simulink model "new68bus_opal"  (R2019b)
settings: Solver=ode4  StartTime=0.0  StopTime=30  FixedStep=Ts  RelTol=1e-3
PreLoadFcn:
  | PSSMODEL=1;
  | LPSS=0;
  | WAPSS=0;
  | WAPSS2=0;
  | Ts=50e-5;
InitFcn:
  | PSSMODEL=1;
  | LPSS=0;
  | WAPSS=0;
  | WAPSS2=0;
  | Ts=50e-5;
  | 
  | % Required data to 68 Bus benchmark
  | % clear
  | % clc
  | % Definition for the columns
  | % system base =100 MVA
  | 
  | %% Line data Format (line)
  | % All values are given on the same system base MVA
  | % 1: From bus
  | % 2: To bus
  | % 3: Resistance (pu)
  | % 4: Reactance  (pu)
  | % 5: Charge     (pu)
  | % 6: Transformer Tap Amplitute
  | % 7: base MVA
  | % 8: Nomonal Voltage (KV)
  | 
  | %1   2    3        4       5       6        7      8
  | line=[...
  | 1	54	0	     0.0181	  0	      1.025     100    13.8
  | 2	58	0	     0.025	  0	      1.070     100    13.8
  | 3	62	0	     0.02	  0	      1.070     100    13.8
  | 4	19	0.0007	 0.0142	  0	      1.070     100    13.8
  | 5	20	0.0009	 0.018	  0	      1.009     100    13.8
  | 6	22	0	     0.0143	  0	      1.025     100    13.8
  | 7	23	0.0005	 0.0272	  0	      0         100    13.8
  | 8	25	0.0006	 0.0232	  0	      1.025     100    13.8
  | 9	29	0.0008	 0.0156   0	      1.025     100    13.8
  | 10	31	0	     0.026	  0	      1.04      100    13.8
  | 11	32	0	     0.013	  0	      1.04      100    13.8
  | 12	36	0	     0.0075	  0	      1.04      100    13.8
  | 13	17	0	     0.0033	  0	      1.04      100    13.8
  | 14	41	0	     0.0015	  0	      1         100    13.8
  | 15	42	0	     0.0015	  0	      1         100    13.8
  | 16	18	0	     0.003	  0	      1         100    13.8
  | 17	36	0.0005	 0.0045	  0.32	  0         100    138
  | 17	43	0.0005	 0.0276	  0	      0         100    138
  | 18	42	0.004	 0.06	  2.25    0         100    138
  | 18	49	0.0076	 0.1141	  1.16    0	        100    138
  | 18	50	0.0012	 0.0288	  2.06	  0         100    138
  | 20	19	0.0007	 0.0138	  0       1.06	    100    138
  | 19	68	0.0016	 0.0195	  0.304	  0         100    138
  | 21	22	0.0008	 0.014	  0.2565  0	        100    138
  | 21	68	0.0008	 0.0135	  0.2548  0	        100    138
  | 22	23	0.0006	 0.0096	  0.1846  0	        100    138
  | 23	24	0.0022	 0.035	  0.361	  0         100    138
  | 24	68	0.0003	 0.0059	  0.068	  0         100    138
  | 25	26	0.0032	 0.0323	  0.531	  0         100    138
  | 25	54	0.007	 0.0086	  0.146	  0         100    138
  | 26	27	0.0014	 0.0147	  0.2396  0	        100    138
  | 26	28	0.0043	 0.0474	  0.7802  0	        100    138
  | 26	29	0.0057	 0.0625	  1.029	  0         100    138
  | 27	37	0.0013	 0.0173	  0.3216  0	        100    138
  | 27	53	0.032	 0.32	  0.41	  0         100    138
  | 29	28	0.0014	 0.0151	  0.249	  0         100    138
  | 30	31	0.0013	 0.0187	  0.333	  0         100    138
  | 30	32	0.0024	 0.0288	  0.488	  0         100    138
  | 30	53	0.0008	 0.0074	  0.48	  0         100    138
  | 30	61	0.00095	 0.00915  0.58	  0         100    138
  | 31	38	0.0011	 0.0147	  0.247	  0         100    138
  | 31	53	0.0016	 0.0163	  0.25	  0         100    138
  | 32	33	0.0008	 0.0099	  0.168	  0         100    138
  | 33	34	0.0011	 0.0157	  0.202	  0         100    138
  | 33	38	0.0036	 0.0444	  0.693	  0         100    138
  | 34	35	0.0001	 0.0074	  0	      0.946     100    138
  | 34	36	0.0033	 0.0111	  1.45	  0         100    138
  | 35	45	0.0007	 0.0175	  1.39	  0         100    138
  | 36	61	0.0011	 0.0098	  0.68	  0         100    138
  | 37	52	0.0007	 0.0082	  0.1319  0	        100    138
  | 37	68	0.0007	 0.0089	  0.1342  0	        100    138
  | 38	46	0.0022	 0.0284	  0.43	  0         100    138
  | 39	44	0	     0.0411	  0	      0         100    138
  | 39	45	0	     0.0839	  0	      0         100    138
  | 40	41	0.006	 0.084	  3.15	  0         100    138
  | 40	48	0.002	 0.022	  1.28	  0         100    138
  | 41	42	0.004	 0.06	  2.25	  0         100    138
  | 43	44	0.0001	 0.0011	  0	      0         100    138
  | 44	45	0.0025	 0.073	  0	      0         100    138
  | 45	51	0.0004	 0.0105	  0.72	  0         100    138
  | 46	49	0.0018	 0.0274	  0.27	  0         100    138
  | 47	48	0.00125	 0.0134	  0.8	  0         100    138
  | 47	53	0.0013	 0.0188	  1.31	  0         100    138
  | 50	51	0.0009	 0.0221	  1.62	  0         100    138
  | 52	55	0.0011	 0.0133	  0.2138  0	        100    138
  | 53	54	0.0035	 0.0411	  0.6987  0	        100    138
  | 54	55	0.0013	 0.0151	  0.2572  0	        100    138
  | 55	56	0.0013	 0.0213	  0.2214  0	        100    138
  | 56	57	0.0008	 0.0128	  0.1342  0	        100    138
  | 56	66	0.0008	 0.0129	  0.1382  0	        100    138
  | 57	58	0.0002	 0.0026	  0.0434  0	        100    138
  | 57	60	0.0008	 0.0112	  0.1476  0	        100    138
  | 58	59	0.0006	 0.0092	  0.113	  0         100    138
  | 58	63	0.0007	 0.0082	  0.1389  0	        100    138
  | 59	60	0.0004	 0.0046	  0.078	  0         100    138
  | 60	61	0.0023	 0.0363	  0.3804  0	        100    138
  | 62	63	0.0004	 0.0043	  0.0729  0	        100    138
  | 62	65	0.0004	 0.0043	  0.0729  0	        100    138
  | 63	64	0.0016	 0.0435	  0	      1.06      100    138
  | 65	64	0.0016	 0.0435	  0	      1.06      100    138
  | 65	66	0.0009	 0.0101	  0.1723  0 	    100    138
  | 66	67	0.0018	 0.0217	  0.366	  0         100    138
  | 67	68	0.0009	 0.0094   0.171   0         100   138 ];
  | 
  | 
  | 
  | %% Power System Stabilizer Format (MB)
  | % Applied power system stabilizer is MBPSS with simplified settings
  | % Note: All machines use MBPSS with same configuration
  | % 1: Global gain (G)
  | % 2: Frequency of low frequency band (FL) Hz
  | % 3: Gain of low frequency band (KL)
  | % 4: Frequency of intermediate frequency band (FI) Hz
  | % 5: Gain of intermediate frequency band (KI)
  | % 6: Frequency of high frequency band (FH) Hz
  | % 7: Gain of high frequency band (KH)
  | %   1    2  3     4   5      6  7
  | MB=[1   0.2 30   1.25 40    12 160];
  | 
  | %% Excitation System format (AVR_Data)
  | % All machines use IEEE type 1 synchronous machine voltage regulator combined to an exciter
  | % 1. Low pass filter time constant (Tr) sec
  | % 2. Regulator gain (Ka)
  | % 3. regulator time constant (Ta) sec
  | % 4. Lead-lag compensator time constant (Tb) sec
  | % 5. Lead-lag compensator time constant (Tc) sec
  | % 6. Terminal voltage (pu)
  | % 7. Lower limit for regulator output (Emin)
  | % 8. Upper limit for regulator output (Emax)
  | %     1    2      3      4     5     6       7    8
  |   AVR_Data=[...
  |     0.01  200    0.015   10    1    1.03    -5    5
  |     0.01  200    0.015   10    1    1.03    -5    5
  |     0.01  200    0.015   10    1    1.03    -5    5
  |     0.01  200    0.015   10    1    1.03    -5    5
  |     0.01  200    0.015   10    1    1.03    -5    5
  |     0.01  200    0.015   10    1    1.03    -5    5
  |     0.01  200    0.015   10    1    1.03    -5    5
  |     0.01  200    0.015   10    1    1.03    -5    5
  |     0.01  200    0.015   10    1    1.03    -5    5
  |     0.01  200    0.015   10    1    1.03    -5    5
  |     0.01  200    0.015   10    1    1.03    -5    5
  |     0.01  200    0.015   10    1    1.03    -5    5
  |     0.01  200    0.015   10    1    1.03    -5    5
  |     0.01  200    0.015   10    1    1.03    -5    5
  |     0.01  200    0.015   10    1    1.03    -5    5
  |     0.01  200    0.015   10    1    1.03    -5    5];
  | 
  | C0=829.7e-9;
  | L0=3.220e-3;
  | R0=1;
  | Ns=120*60/(2); %Nominal speed of synchronous machines
  | s=10;
  | 
  | %% Machine Data Format (mac_con)
  | % 1.  Machine Number
  | % 2.  Bus Number
  | % 3.  Base MVA
  | % 4.  Leakage Reactance x_l(pu)
  | % 5.  Resistance r_a(pu)
  | % 6.  d-axis sychronous reactance x_d(pu)
  | % 7.  d-axis transient reactance x'_d(pu)
  | % 8.  d-axis subtransient reactance x"_d(pu)
  | % 9.  d-axis open-circuit time constant T'_do(sec),
  | % 10. d-axis open-circuit subtransient time constant T"_do(sec)
  | % 11. q-axis sychronous reactance x_q(pu)
  | % 12. q-axis transient reactance x'_q(pu)
  | % 13. q-axis subtransient reactance x"_q(pu)
  | % 14. q-axis open-circuit time constant T'_qo(sec)
  | % 15. q-axis open circuit subtransient time constant % T"_qo(sec)
  | % 16. inertia constant H(sec)
  | % 17. damping coefficient d_o(pu)
  | % 18. dampling coefficient d_1(pu)
  | % 19. bus number
  | % Note: all the following machines use sub-transient model
  | % 1  2     3      4      5     6     7    8      9    10    11    12    13    14    15    16    17    18  19
  | mac_con = [ 01 01 100 0.0125 0.0 0.1 0.031 0.025 10.2 0.05 0.069 0.0416667 0.025 1.5 0.035 42. 0 0 01 0 0; 02 02 100 0.035 0.0 0.295 0.0697 0.05 6.56 0.05 0.282 0.0933333 0.05 1.5 0.035 30.2 0 0 02 0 0; 03 03 100 0.0304 0.0 0.2495 0.0531 0.045 5.7 0.05 0.237 0.0714286 0.045 1.5 0.035 35.8 0 0 03 0 0; 04 04 100 0.0295 0.0 0.262 0.0436 0.035 5.69 0.05 0.258 0.0585714 0.035 1.5 0.035 28.6 0 0 04 0 0; 05 05 100 0.027 0.0 0.33 0.066 0.05 5.4 0.05 0.31 0.0883333 0.05 0.44 0.035 26. 0 0 05 0 0; 06 06 100 0.0224 0.0 0.254 0.05 0.04 7.3 0.05 0.241 0.0675000 0.04 0.4 0.035 34.8 0 0 06 0 0; 07 07 100 0.0322 0.0 0.295 0.049 0.04 5.66 0.05 0.292 0.0666667 0.04 1.5 0.035 26.4 0 0 07 0 0; 08 08 100 0.028 0.0 0.29 0.057 0.045 6.7 0.05 0.280 0.0766667 0.045 0.41 0.035 24.3 0 0 08 0 0; 09 09 100 0.0298 0.0 0.2106 0.057 0.045 4.79 0.05 0.205 0.0766667 0.045 1.96 0.035 34.5 0 0 09 0 0; 10 10 100 0.0199 0.0 0.169 0.0457 0.04 9.37 0.05 0.115 0.0615385 0.04 1.5 0.035 31.0 0 0 10 0 0; 11 11 100 0.0103 0.0 0.128 0.018 0.012 4.1 0.05 0.123 0.0241176 0.012 1.5 0.035 28.2 0 0 11 0 0; 12 12 100 0.022 0.0 0.101 0.031 0.025 7.4 0.05 0.095 0.0420000 0.025 1.5 0.035 92.3 0 0 12 0 0; 13 13 200 0.0030 0.0 0.0296 0.0055 0.004 5.9 0.05 0.0286 0.0074000 0.004 1.5 0.035 248.0 0 0 13 0 0; 14 14 100 0.0017 0.0 0.018 0.00285 0.0023 4.1 0.05 0.0173 0.0037931 0.0023 1.5 0.035 300.0 0 0 14 0 0; 15 15 100 0.0017 0.0 0.018 0.00285 0.0023 4.1 0.05 0.0173 0.0037931 0.0023 1.5 0.035 300.0 0 0 15 0 0; 16 16 200 0.0041 0.0 0.0356 0.0071 0.0055 7.8 0.05 0.0334 0.0095000 0.0055 1.5 0.035 225.0 0 0 16 0 0; ] ;
  | 
  | p0=[250/200 545/200 650/200 632/200 505/200 700/200 560/200 540/200 800/200 500/200 1000/200 1350/200 3591/6000 1785/3000 1000/3000 3379.57/6000];%'./1000;%Active Power Generation of PV units
  | Pn(1:16,1)=1; % Nominal Power
  | % PSSModel=1;%1:No pSS //1:MB
  | %% Bus data (Bus)
  | % 1. Bus number
  | % 2. Nominal phase-phase voltage
  | %    1    2
  | Bus = [ ...
  | 1	13.8
  | 2	13.8
  | 3	13.8
  | 4	13.8
  | 5	13.8
  | 6	13.8
  | 7	13.8
  | 8	13.8
  | 9	13.8
  | 10	13.8
  | 11	13.8
  | 12	13.8
  | 13	13.8
  | 14	13.8
  | 15	13.8
  | 16	13.8
  | 17	138
  | 18	138
  | 19	138
  | 20	138
  | 21	138
  | 22	138
  | 23	138
  | 24	138
  | 25	138
  | 26	138
  | 27	138
  | 28	138
  | 29	138
  | 30	138
  | 31	138
  | 32	138
  | 33	138
  | 34	138
  | 35	138
  | 36	138
  | 37	138
  | 38	138
  | 39	138
  | 40	138
  | 41	138
  | 42	138
  | 43	138
  | 44	138
  | 45	138
  | 46	138
  | 47	138
  | 48	138
  | 49	138
  | 50	138
  | 51	138
  | 52	138
  | 53	138
  | 54	138
  | 55	138
  | 56	138
  | 57	138
  | 58	138
  | 59	138
  | 60	138
  | 61	138
  | 62	138
  | 63	138
  | 64	138
  | 65	138
  | 66	138
  | 67	138
  | 68	138];
  | 
  |    zbase=(line(:,8).^2)./line(:,7);
  |    line(:,3)=line(:,3).*zbase;
  |    line(:,4)=line(:,4).*zbase/(120*pi);
  |    line(:,5)=line(:,5)./zbase/(120*pi);
  | 
  | %PSSMODEL=1;
undefined symbols (not defined in the file or in its folder): D1, Delta, I, Left, Right, type, V
libraries: powerlib x359, artemis x26, sps_avr x16, powerlib_meascontrol x5, rtlab x1
(part 1 of 8)
settings Model: ARTEMISmethode_block_infos=$$__separator__$$new68bus_opal/ARTEMIS Guide$$__separator__$$  Creator=rubai  LastModifiedBy=shamim

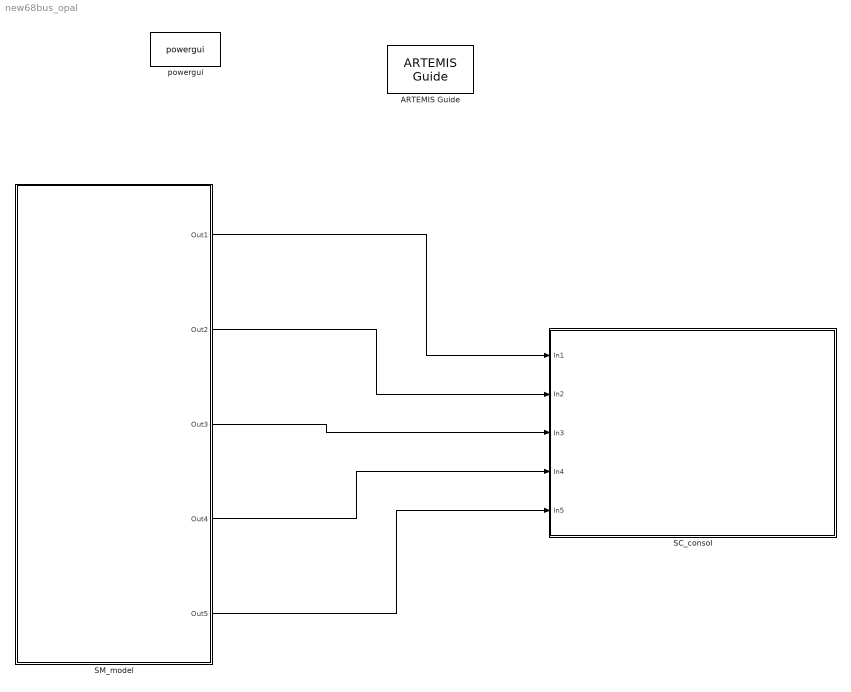
== system new68bus_opal ==
  ARTEMIS Guide : artemis/ARTEMIS/ARTEMIS Guide  Tag=art7.5  Description=New ARTEMiS block v 7.5b (R2015b+)  lock=on  Ts=Ts  ssn=on  opt=art5  dyna=off  nb_perm=4  RT_fullcomp=off  ssn_itvc=off  ssn_ivic=off  ssn_ext=off  ssn_solver=Art5  iter_type=iSWITCH and iMOV only (default)  ssn_ImpulseLoopBlockedStateUpdate=5  ssn_mov_iter_number=5  ssn_switch_iter_number=3  ssn_lu_or_ldlt=LU (more robust)  ssn_nib_type_verify=off  ssn_use_lu=on  ssn_use_ldlt=off  ssn_impulse=on  ssn_quasimpulse=off  ssn_impulse_loop=5  paraExtinctionThy=off  Thy_Impulse=on  dtc=Off  dtc_opt=normal  ao=off  simtype=off  ct_mac=off  lin_mov=off  lsp=[0.001 2]  spike_skip=Disabled  dtc_extra=1  dtc_sws=normal  dtc_pied=0.5  SPSRulesBlock=SPSRules  tre=off  ctmm=off  LF=off  dpl_type=ARTEMiS DPL  rlc_type=off  custom_type=off  para=on  ssn_full_iteration=off
  SC_consol : Subsystem
  SM_model : Subsystem
  powergui : powerlib/powergui  Priority=1  SimulationMode=Discrete  SampleTime=Ts  frequency=60  Iterations=50  frequencyindice=60  Pbase=100e6  ErrMax=1e-4  UnitsV=kV  UnitsW=MW  buscounter=0  FunctionMessages=off  echomessages=off  EnableUseOfTLC=off  CurrentSourceSwitches=off  DisableSnubberDevices=off  DisableRonSwitches=off  DisableVfSwitches=off  DisplayEquations=off  AutomaticDiscreteSolvers=on  SolverType=Tustin/Backward Euler (TBE)  Interpol=off  ExternalGateDelay=off  methode=off  Ts=100  x0status=blocks  SPID=on  SwTol=0  HookPort=off  NonlinearTolerance=1e-4  nMaxIteration=100  ContinueOnMaxIteration=off  RestoreLinks=warning  ResistiveCurrentMeasurement=off  Frange=[0:2:500]  Ylog=off  Xlog=on  ShowGrid=off  save=off  variable=ZData  structure=0  ZoomFFT=off  StartTime=0.0  cycles=1  DisplayStyle=1  fundamental=60  FreqAxis=off  MaxFrequency=1000  frequencyindicesteady=1  RmsSteady=1  display=off
      settings: SourceProductName=Simscape Electrical
  wires:
  SM_model/1(Out1) -> SC_consol/1(In1)
  SM_model/2(Out2) -> SC_consol/2(In2)
  SM_model/3(Out3) -> SC_consol/3(In3)
  SM_model/4(Out4) -> SC_consol/4(In4)
  SM_model/5(Out5) -> SC_consol/5(In5)

== system new68bus_opal/SC_consol ==
  In1 : Inport
  In2 : Inport  Port=2
  In3 : Inport  Port=3
  In4 : Inport  Port=4
  In5 : Inport  Port=5
  Display : Display
  OpComm : rtlab/OpComm  nbport=5  groupe_acq=1  subsys_rate=0  st=0  Synchronization=off  Interpolation=off  Threshold=1.0  Missed_Data=off  Sim_Time=off  Samples=off  dynSigOut=off  from_console=0  warning_done=off  writeOpCommFile=off  Offset=off
      settings: SourceProductName=RT-LAB
  Scope{,1..4} (5 alike) : Scope
  wires:
  In2/1 -> OpComm/2
  In5/1 -> OpComm/5
  In3/1 -> OpComm/3
  OpComm/1 -> Scope/1
  OpComm/2 -> Display/1, Scope1/1
  OpComm/3 -> Scope2/1
  In4/1 -> OpComm/4
  OpComm/5 -> Scope4/1
  OpComm/4 -> Scope3/1
  In1/1 -> OpComm/1

== system new68bus_opal/SM_model ==
  20-1 : powerlib/Elements/Three-Phase PI Section Line  LConnTagsString=a|b|c  RConnTagsString=A|B|C  Frequency=60  Resistances=[line(20,3) 3*line(20,3)]  Inductances=[line(20,4) 3*line(20,4)]  Capacitances=[line(20,5) line(20,5)/3]  Length=1
      settings: SourceProductName=Simscape Electrical
  21-1 : powerlib/Elements/Three-Phase PI Section Line  LConnTagsString=a|b|c  RConnTagsString=A|B|C  Frequency=60  Resistances=[line(21,3) 3*line(21,3)]  Inductances=[line(21,4) 3*line(21,4)]  Capacitances=[line(21,5) line(21,5)/3]  Length=1
      settings: SourceProductName=Simscape Electrical
  34-1 : powerlib/Elements/Three-Phase PI Section Line  LConnTagsString=a|b|c  RConnTagsString=A|B|C  Frequency=60  Resistances=[line(34,3) 3*line(34,3)]  Inductances=[line(34,4) 3*line(34,4)]  Capacitances=[line(34,5) line(34,5)/3]  Length=1
      settings: SourceProductName=Simscape Electrical
  39-1 : powerlib/Elements/Three-Phase PI Section Line  LConnTagsString=a|b|c  RConnTagsString=A|B|C  Frequency=60  Resistances=[line(39,3) 3*line(39,3)]  Inductances=[line(39,4) 3*line(39,4)]  Capacitances=[line(39,5) line(39,5)/3]  Length=1
      settings: SourceProductName=Simscape Electrical
  42-1 : powerlib/Elements/Three-Phase PI Section Line  LConnTagsString=a|b|c  RConnTagsString=A|B|C  Frequency=60  Resistances=[line(42,3) 3*line(42,3)]  Inductances=[line(42,4) 3*line(42,4)]  Capacitances=[line(42,5) line(42,5)/3]  Length=1
      settings: SourceProductName=Simscape Electrical
  51-1 : powerlib/Elements/Three-Phase PI Section Line  LConnTagsString=a|b|c  RConnTagsString=A|B|C  Frequency=60  Resistances=[line(51,3) 3*line(51,3)]  Inductances=[line(51,4) 3*line(51,4)]  Capacitances=[line(51,5) line(51,5)/3]  Length=1
      settings: SourceProductName=Simscape Electrical
  62-1 : powerlib/Elements/Three-Phase PI Section Line  LConnTagsString=a|b|c  RConnTagsString=A|B|C  Frequency=60  Resistances=[line(62,3) 3*line(62,3)]  Inductances=[line(62,4) 3*line(62,4)]  Capacitances=[line(62,5) line(62,5)/3]  Length=1
      settings: SourceProductName=Simscape Electrical
  67-1 : powerlib/Elements/Three-Phase PI Section Line  LConnTagsString=a|b|c  RConnTagsString=A|B|C  Frequency=60  Resistances=[line(67,3) 3*line(67,3)]  Inductances=[line(67,4) 3*line(67,4)]  Capacitances="[line(67,5)  line(67,5)/3]"  Length=1
      settings: SourceProductName=Simscape Electrical
  76-1 : powerlib/Elements/Three-Phase PI Section Line  LConnTagsString=a|b|c  RConnTagsString=A|B|C  Frequency=60  Resistances=[line(76,3) 3*line(76,3)]  Inductances=[line(76,4) 3*line(76,4)]  Capacitances=[line(76,5) line(76,5)/3]  Length=1
      settings: SourceProductName=Simscape Electrical
  83-1 : powerlib/Elements/Three-Phase PI Section Line  LConnTagsString=a|b|c  RConnTagsString=A|B|C  Frequency=60  Resistances=[line(83,3) 3*line(83,3)]  Inductances=[line(83,4) 3*line(83,4)]  Capacitances=[line(83,5) line(83,5)/3]  Length=1
      settings: SourceProductName=Simscape Electrical
  "Bus Voltages " : Subsystem  Commented=on
  PSS model : Constant  Value=PSSMODEL
  SSN Interface Block (3ph) : artemis/SSN/Nodal Interface Blocks/SSN Interface Block (3ph)  nb_phase=3  nb_port=2  p1_type=I-type(Left)  p2_type=I-type(Right)  p3_type=V-type(Left)  p4_type=V-type(Left)  p5_type=V-type(Left)  p6_type=V-type(Left)  p7_type=V-type(Left)  p8_type=V-type(Left)  p9_type=V-type(Left)  p10_type=V-type(Left)  p11_type=V-type(Left)  p12_type=V-type(Left)  p13_type=V-type(Left)  p14_type=V-type(Left)  p15_type=V-type(Left)  p16_type=V-type(Left)  I_port_shunt_resistance=1e9
  SSN group tag : artemis/SSN/SSN group tag  ssn_group_tag=ssn2a
  SSN group tag1 : artemis/SSN/SSN group tag  ssn_group_tag=ssn2b
  Subsystem : Subsystem
  area-1 : Subsystem
  area-2 : Subsystem
  area-3 : Subsystem
  area-4 : Subsystem
  "voltage measurement " : Subsystem
  Out1 : Outport
  Out2 : Outport  Port=2
  Out3 : Outport  Port=3
  Out4 : Outport  Port=4
  Out5 : Outport  Port=5
  tag scope: PSSmodel=global
  wires:
  "voltage measurement "/2(Output1) -> Out2/1
  "voltage measurement "/4(Output3) -> Out4/1
  "voltage measurement "/3(Output2) -> Out3/1
  PSS model/1 -> [PSSmodel]
  "voltage measurement "/1(Output) -> Out1/1
  "voltage measurement "/5(Output4) -> Out5/1
  connections:
  62-1/LConn3 -- area-3/RConn12
  62-1/RConn1 -- Subsystem/RConn5
  21-1/LConn3 -- area-4/RConn15
  51-1/LConn2 -- area-2/RConn6
  67-1/RConn1 -- area-3/RConn4
  83-1/LConn3 -- area-2/RConn3
  Subsystem/RConn2 -- 21-1/RConn2 -- 20-1/RConn2
  67-1/RConn3 -- area-3/RConn6
  42-1/LConn1 -- area-3/RConn7
  42-1/RConn2 -- area-4/RConn5
  62-1/RConn3 -- Subsystem/RConn6
  Subsystem/RConn3 -- 21-1/RConn3 -- 20-1/RConn3
  67-1/LConn3 -- area-2/RConn9
  62-1/RConn2 -- Subsystem/RConn4
  67-1/LConn2 -- area-2/RConn8
  62-1/LConn1 -- area-3/RConn10
  area-2/RConn14 -- 34-1/RConn2
  76-1/LConn2 -- area-4/RConn11
  42-1/LConn2 -- area-3/RConn8
  51-1/LConn1 -- area-2/RConn4
  42-1/LConn3 -- area-3/RConn9
  83-1/RConn1 -- SSN Interface Block (3ph)/RConn1 -- 51-1/RConn1
  42-1/RConn1 -- area-4/RConn4
  76-1/RConn3 -- area-2/RConn12
  area-3/RConn2 -- 34-1/LConn2
  21-1/LConn1 -- area-4/RConn13
  39-1/LConn3 -- area-4/RConn9
  area-2/RConn13 -- 34-1/RConn1
  67-1/LConn1 -- area-2/RConn7
  76-1/RConn2 -- area-2/RConn11
  21-1/LConn2 -- area-4/RConn14
  area-2/RConn15 -- 34-1/RConn3
  83-1/RConn3 -- SSN group tag1/LConn1 -- SSN Interface Block (3ph)/RConn3 -- 51-1/RConn3
  area-2/RConn5 -- 51-1/LConn3
  39-1/RConn2 -- area-3/RConn14
  42-1/RConn3 -- area-4/RConn6
  20-1/LConn2 -- area-4/RConn2
  area-3/RConn1 -- 34-1/LConn1
  76-1/RConn1 -- area-2/RConn10
  76-1/LConn1 -- area-4/RConn10
  39-1/RConn1 -- area-3/RConn15
  67-1/RConn2 -- area-3/RConn5
  83-1/LConn1 -- area-2/RConn1
  20-1/LConn3 -- area-4/RConn3
  83-1/LConn2 -- area-2/RConn2
  39-1/LConn1 -- area-4/RConn7
  39-1/RConn3 -- area-3/RConn13
  83-1/RConn2 -- SSN Interface Block (3ph)/RConn2 -- 51-1/RConn2
  Subsystem/RConn1 -- 21-1/RConn1 -- 20-1/RConn1
  39-1/LConn2 -- area-4/RConn8
  area-3/RConn3 -- 34-1/LConn3
  20-1/LConn1 -- area-4/RConn1
  62-1/LConn2 -- area-3/RConn11
  76-1/LConn3 -- area-4/RConn12
  SSN Interface Block (3ph)/LConn1 -- area-1/RConn1
  SSN Interface Block (3ph)/LConn2 -- area-1/RConn2
  SSN Interface Block (3ph)/LConn3 -- SSN group tag/LConn1 -- area-1/RConn3

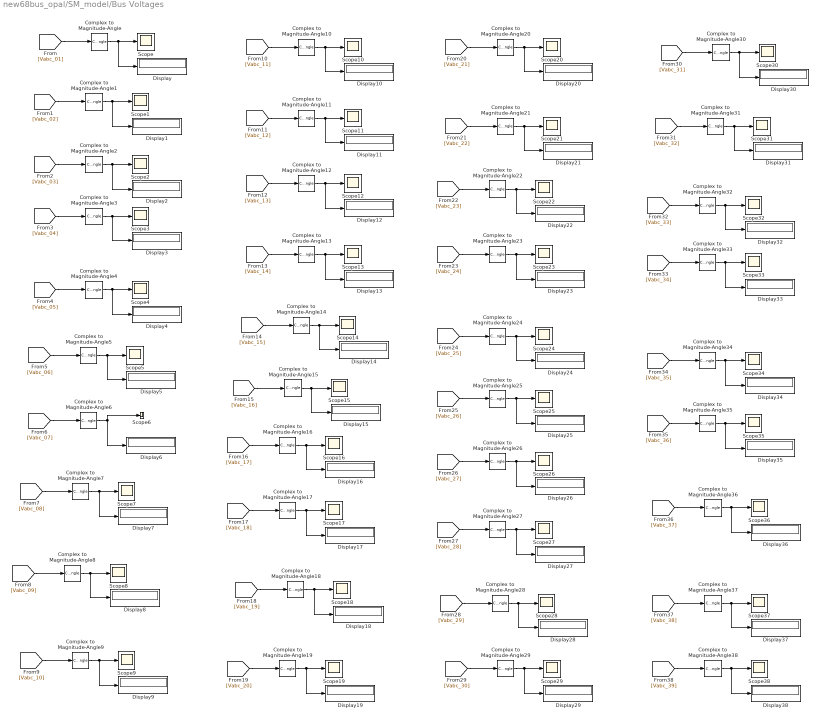
== system new68bus_opal/SM_model/Bus Voltages  ==
  Complex to Magnitude-Angle{,1..38} (39 alike) : ComplexToMagnitudeAngle  Output=Magnitude
  Display{,1..38} (39 alike) : Display
  Scope{,1..38} (39 alike) : Scope
  wires:
  [Vabc_01] -> Complex to Magnitude-Angle/1
  Complex to Magnitude-Angle/1 -> Display/1, Scope/1
  [Vabc_02] -> Complex to Magnitude-Angle1/1
  Complex to Magnitude-Angle1/1 -> Display1/1, Scope1/1
  [Vabc_03] -> Complex to Magnitude-Angle2/1
  Complex to Magnitude-Angle2/1 -> Display2/1, Scope2/1
  [Vabc_04] -> Complex to Magnitude-Angle3/1
  Complex to Magnitude-Angle3/1 -> Display3/1, Scope3/1
  [Vabc_05] -> Complex to Magnitude-Angle4/1
  Complex to Magnitude-Angle4/1 -> Display4/1, Scope4/1
  [Vabc_06] -> Complex to Magnitude-Angle5/1
  Complex to Magnitude-Angle5/1 -> Display5/1, Scope5/1
  [Vabc_07] -> Complex to Magnitude-Angle6/1
  Complex to Magnitude-Angle6/1 -> Display6/1, Scope6/1
  [Vabc_08] -> Complex to Magnitude-Angle7/1
  Complex to Magnitude-Angle7/1 -> Display7/1, Scope7/1
  [Vabc_09] -> Complex to Magnitude-Angle8/1
  Complex to Magnitude-Angle8/1 -> Display8/1, Scope8/1
  [Vabc_10] -> Complex to Magnitude-Angle9/1
  Complex to Magnitude-Angle9/1 -> Display9/1, Scope9/1
  [Vabc_11] -> Complex to Magnitude-Angle10/1
  Complex to Magnitude-Angle10/1 -> Display10/1, Scope10/1
  [Vabc_12] -> Complex to Magnitude-Angle11/1
  Complex to Magnitude-Angle11/1 -> Display11/1, Scope11/1
  [Vabc_13] -> Complex to Magnitude-Angle12/1
  Complex to Magnitude-Angle12/1 -> Display12/1, Scope12/1
  [Vabc_14] -> Complex to Magnitude-Angle13/1
  Complex to Magnitude-Angle13/1 -> Display13/1, Scope13/1
  [Vabc_15] -> Complex to Magnitude-Angle14/1
  Complex to Magnitude-Angle14/1 -> Display14/1, Scope14/1
  Complex to Magnitude-Angle15/1 -> Scope15/1, Display15/1
  [Vabc_16] -> Complex to Magnitude-Angle15/1
  [Vabc_17] -> Complex to Magnitude-Angle16/1
  Complex to Magnitude-Angle16/1 -> Display16/1, Scope16/1
  Complex to Magnitude-Angle17/1 -> Scope17/1, Display17/1
  [Vabc_18] -> Complex to Magnitude-Angle17/1
  [Vabc_19] -> Complex to Magnitude-Angle18/1
  Complex to Magnitude-Angle18/1 -> Display18/1, Scope18/1
  Complex to Magnitude-Angle19/1 -> Scope19/1, Display19/1
  [Vabc_20] -> Complex to Magnitude-Angle19/1
  Complex to Magnitude-Angle20/1 -> Scope20/1, Display20/1
  [Vabc_21] -> Complex to Magnitude-Angle20/1
  [Vabc_22] -> Complex to Magnitude-Angle21/1
  Complex to Magnitude-Angle21/1 -> Display21/1, Scope21/1
  Complex to Magnitude-Angle22/1 -> Scope22/1, Display22/1
  [Vabc_23] -> Complex to Magnitude-Angle22/1
  [Vabc_24] -> Complex to Magnitude-Angle23/1
  Complex to Magnitude-Angle23/1 -> Display23/1, Scope23/1
  Complex to Magnitude-Angle24/1 -> Scope24/1, Display24/1
  [Vabc_25] -> Complex to Magnitude-Angle24/1
  [Vabc_26] -> Complex to Magnitude-Angle25/1
  Complex to Magnitude-Angle25/1 -> Display25/1, Scope25/1
  Complex to Magnitude-Angle26/1 -> Scope26/1, Display26/1
  [Vabc_27] -> Complex to Magnitude-Angle26/1
  [Vabc_28] -> Complex to Magnitude-Angle27/1
  Complex to Magnitude-Angle27/1 -> Display27/1, Scope27/1
  Complex to Magnitude-Angle28/1 -> Scope28/1, Display28/1
  [Vabc_29] -> Complex to Magnitude-Angle28/1
  [Vabc_30] -> Complex to Magnitude-Angle29/1
  Complex to Magnitude-Angle29/1 -> Display29/1, Scope29/1
  Complex to Magnitude-Angle30/1 -> Scope30/1, Display30/1
  [Vabc_31] -> Complex to Magnitude-Angle30/1
  [Vabc_32] -> Complex to Magnitude-Angle31/1
  Complex to Magnitude-Angle31/1 -> Display31/1, Scope31/1
  Complex to Magnitude-Angle32/1 -> Scope32/1, Display32/1
  [Vabc_33] -> Complex to Magnitude-Angle32/1
  [Vabc_34] -> Complex to Magnitude-Angle33/1
  Complex to Magnitude-Angle33/1 -> Display33/1, Scope33/1
  Complex to Magnitude-Angle34/1 -> Scope34/1, Display34/1
  [Vabc_35] -> Complex to Magnitude-Angle34/1
  [Vabc_36] -> Complex to Magnitude-Angle35/1
  Complex to Magnitude-Angle35/1 -> Display35/1, Scope35/1
  Complex to Magnitude-Angle36/1 -> Scope36/1, Display36/1
  [Vabc_37] -> Complex to Magnitude-Angle36/1
  [Vabc_38] -> Complex to Magnitude-Angle37/1
  Complex to Magnitude-Angle37/1 -> Display37/1, Scope37/1
  Complex to Magnitude-Angle38/1 -> Scope38/1, Display38/1
  [Vabc_39] -> Complex to Magnitude-Angle38/1

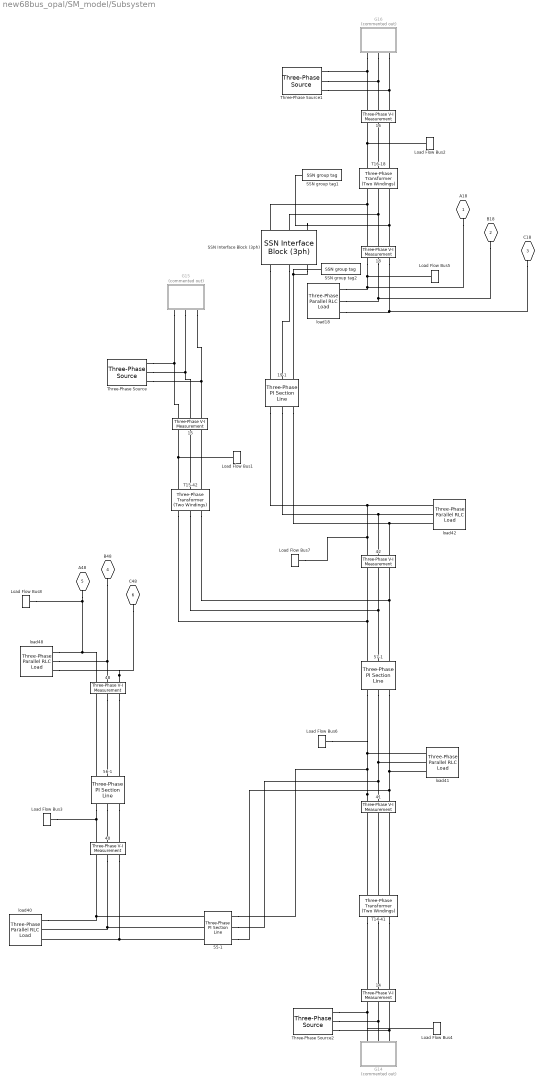
== system new68bus_opal/SM_model/Subsystem ==
  14 : powerlib/Measurements/Three-Phase V-I Measurement  VoltageMeasurement=phase-to-phase  SetLabelV=on  LabelV=Vabc_14  Vpu=off  VpuLL=on  CurrentMeasurement=no  SetLabelI=off  LabelI=Iabc  Ipu=off  Pbase=100e6  Vbase=13.8e3  OutputType=Complex  PhasorSimulation=off  PSBequivalent=0
      settings: SourceProductName=Simscape Electrical
  15 : powerlib/Measurements/Three-Phase V-I Measurement  VoltageMeasurement=phase-to-phase  SetLabelV=on  LabelV=Vabc_15  Vpu=off  VpuLL=on  CurrentMeasurement=no  SetLabelI=off  LabelI=Iabc  Ipu=off  Pbase=100e6  Vbase=13.8e3  OutputType=Complex  PhasorSimulation=off  PSBequivalent=0
      settings: SourceProductName=Simscape Electrical
  16 : powerlib/Measurements/Three-Phase V-I Measurement  VoltageMeasurement=phase-to-phase  SetLabelV=on  LabelV=Vabc_16  Vpu=off  VpuLL=on  CurrentMeasurement=no  SetLabelI=off  LabelI=Iabc  Ipu=off  Pbase=100e6  Vbase=13.8e3  OutputType=Complex  PhasorSimulation=off  PSBequivalent=0
      settings: SourceProductName=Simscape Electrical
  18 : powerlib/Measurements/Three-Phase V-I Measurement  VoltageMeasurement=phase-to-phase  SetLabelV=on  LabelV=Vabc_18  Vpu=off  VpuLL=on  CurrentMeasurement=no  SetLabelI=off  LabelI=Iabc  Ipu=off  Pbase=100e6  Vbase=Bus(18,2)*1e3  OutputType=Complex  PhasorSimulation=off  PSBequivalent=0
      settings: SourceProductName=Simscape Electrical
  19-1 : powerlib/Elements/Three-Phase PI Section Line  LConnTagsString=a|b|c  RConnTagsString=A|B|C  Frequency=60  Resistances=[line(19,3) 3*line(19,3)]  Inductances=[line(19,4) 3*line(19,4)]  Capacitances=[line(19,5) line(19,5)/3]  Length=1
      settings: SourceProductName=Simscape Electrical
  40 : powerlib/Measurements/Three-Phase V-I Measurement  VoltageMeasurement=phase-to-phase  SetLabelV=on  LabelV=Vabc_40  Vpu=off  VpuLL=on  CurrentMeasurement=no  SetLabelI=off  LabelI=Iabc  Ipu=off  Pbase=100e6  Vbase=Bus(40,2)*1e3  OutputType=Complex  PhasorSimulation=off  PSBequivalent=0
      settings: SourceProductName=Simscape Electrical
  41 : powerlib/Measurements/Three-Phase V-I Measurement  VoltageMeasurement=phase-to-phase  SetLabelV=on  LabelV=Vabc_41  Vpu=off  VpuLL=on  CurrentMeasurement=no  SetLabelI=off  LabelI=Iabc  Ipu=off  Pbase=100e6  Vbase=Bus(41,2)*1e3  OutputType=Complex  PhasorSimulation=off  PSBequivalent=0
      settings: SourceProductName=Simscape Electrical
  42 : powerlib/Measurements/Three-Phase V-I Measurement  VoltageMeasurement=phase-to-phase  SetLabelV=on  LabelV=Vabc_42  Vpu=off  VpuLL=on  CurrentMeasurement=no  SetLabelI=off  LabelI=Iabc  Ipu=off  Pbase=100e6  Vbase=Bus(42,2)*1e3  OutputType=Complex  PhasorSimulation=off  PSBequivalent=0
      settings: SourceProductName=Simscape Electrical
  48 : powerlib/Measurements/Three-Phase V-I Measurement  VoltageMeasurement=phase-to-phase  SetLabelV=on  LabelV=Vabc_48  Vpu=off  VpuLL=on  CurrentMeasurement=no  SetLabelI=off  LabelI=Iabc  Ipu=off  Pbase=100e6  Vbase=Bus(48,2)*1e3  OutputType=Complex  PhasorSimulation=off  PSBequivalent=0
      settings: SourceProductName=Simscape Electrical
  55-1 : powerlib/Elements/Three-Phase PI Section Line  LConnTagsString=a|b|c  RConnTagsString=A|B|C  Frequency=60  Resistances=[line(55,3) 3*line(55,3)]  Inductances=[line(55,4) 3*line(55,4)]  Capacitances=[line(55,5) line(55,5)/3]  Length=1
      settings: SourceProductName=Simscape Electrical
  56-1 : powerlib/Elements/Three-Phase PI Section Line  LConnTagsString=a|b|c  RConnTagsString=A|B|C  Frequency=60  Resistances=[line(56,3) 3*line(56,3)]  Inductances=[line(56,4) 3*line(56,4)]  Capacitances=[line(56,5) line(56,5)/3]  Length=1
      settings: SourceProductName=Simscape Electrical
  57-1 : powerlib/Elements/Three-Phase PI Section Line  LConnTagsString=a|b|c  RConnTagsString=A|B|C  Frequency=60  Resistances=[line(57,3) 3*line(57,3)]  Inductances=[line(57,4) 3*line(57,4)]  Capacitances=[line(57,5) line(57,5)/3]  Length=1
      settings: SourceProductName=Simscape Electrical
  G14 : Subsystem  Commented=on
  G15 : Subsystem  Commented=on
  G16 : Subsystem  Commented=on
  Load Flow Bus1 : powerlib/Measurements/Load Flow Bus  LConnTagsString=a  Phases=single  Connectors=on one side  ID=BUS_15  Vbase=13.8e3  Vref=1  Vangle=0  VLF=1  VLFb=1  VLFc=1  angleLF=0  angleLFb=0  angleLFc=0
      settings: SourceProductName=Simscape Electrical
  Load Flow Bus2 : powerlib/Measurements/Load Flow Bus  LConnTagsString=a  Phases=single  Connectors=on one side  ID=BUS_16  Vbase=13.8e3  Vref=1  Vangle=0  VLF=1  VLFb=1  VLFc=1  angleLF=0  angleLFb=0  angleLFc=0
      settings: SourceProductName=Simscape Electrical
  Load Flow Bus3 : powerlib/Measurements/Load Flow Bus  LConnTagsString=a  Phases=single  Connectors=on one side  ID=BUS_40  Vbase=138e3  Vref=1  Vangle=0  VLF=1  VLFb=1  VLFc=1  angleLF=0  angleLFb=0  angleLFc=0
      settings: SourceProductName=Simscape Electrical
  Load Flow Bus4 : powerlib/Measurements/Load Flow Bus  LConnTagsString=a  Phases=single  Connectors=on one side  ID=BUS_14  Vbase=13.8e3  Vref=1  Vangle=0  VLF=1  VLFb=1  VLFc=1  angleLF=0  angleLFb=0  angleLFc=0
      settings: SourceProductName=Simscape Electrical
  Load Flow Bus5 : powerlib/Measurements/Load Flow Bus  LConnTagsString=a  Phases=single  Connectors=on one side  ID=BUS_18  Vbase=138e3  Vref=1  Vangle=0  VLF=1  VLFb=1  VLFc=1  angleLF=0  angleLFb=0  angleLFc=0
      settings: SourceProductName=Simscape Electrical
  Load Flow Bus6 : powerlib/Measurements/Load Flow Bus  LConnTagsString=a  Phases=single  Connectors=on one side  ID=BUS_41  Vbase=138e3  Vref=1  Vangle=0  VLF=1  VLFb=1  VLFc=1  angleLF=0  angleLFb=0  angleLFc=0
      settings: SourceProductName=Simscape Electrical
  Load Flow Bus7 : powerlib/Measurements/Load Flow Bus  LConnTagsString=a  Phases=single  Connectors=on one side  ID=BUS_42  Vbase=138e3  Vref=1  Vangle=0  VLF=1  VLFb=1  VLFc=1  angleLF=0  angleLFb=0  angleLFc=0
      settings: SourceProductName=Simscape Electrical
  Load Flow Bus8 : powerlib/Measurements/Load Flow Bus  LConnTagsString=a  Phases=single  Connectors=on one side  ID=BUS_48  Vbase=138e3  Vref=1  Vangle=0  VLF=1  VLFb=1  VLFc=1  angleLF=0  angleLFb=0  angleLFc=0
      settings: SourceProductName=Simscape Electrical
  SSN Interface Block (3ph) : artemis/SSN/Nodal Interface Blocks/SSN Interface Block (3ph)  nb_phase=3  nb_port=2  p1_type=I-type(Left)  p2_type=I-type(Right)  p3_type=V-type(Left)  p4_type=V-type(Left)  p5_type=V-type(Left)  p6_type=V-type(Left)  p7_type=V-type(Left)  p8_type=V-type(Left)  p9_type=V-type(Left)  p10_type=V-type(Left)  p11_type=V-type(Left)  p12_type=V-type(Left)  p13_type=V-type(Left)  p14_type=V-type(Left)  p15_type=V-type(Left)  p16_type=V-type(Left)  I_port_shunt_resistance=1e9
  SSN group tag1 : artemis/SSN/SSN group tag  ssn_group_tag=ssn4a
  SSN group tag2 : artemis/SSN/SSN group tag  ssn_group_tag=ssn4b
  T14-41 : powerlib/Elements/Three-Phase Transformer (Two Windings)  Winding1Connection=Delta (D1)  Winding2Connection=Yg  CoreType=Three single-phase transformers  SetSaturation=off  Hysteresis=off  DataFile='hysteresis'  SetInitialFlux=off  Measurements=None  UNITS=pu  NominalPower=[ 10000e6 , 60 ]  Winding1=[ 13.8e3 , 0.0 , 0 ]  Winding2=[ 138e3 , 0.0 , 0.0015 ]  Rm=500  Lm=500  L0=0.5  Saturation=[ 0,0 ; 0.0024,1.2 ; 1.0,1.52 ]  InitialFluxes=[ 0.8 , -0.8 , 0.7 ]  BreakLoop=off  DiscreteSolver=Trapezoidal robust  DataType=off  TransfoNumber=1
      settings: SourceProductName=Simscape Electrical
  T15-42 : powerlib/Elements/Three-Phase Transformer (Two Windings)  Winding1Connection=Delta (D1)  Winding2Connection=Yg  CoreType=Three single-phase transformers  SetSaturation=off  Hysteresis=off  DataFile='hysteresis'  SetInitialFlux=off  Measurements=None  UNITS=pu  NominalPower=[ 10000e6 , 60 ]  Winding1=[ 13.8e3 , 0.0 , 0 ]  Winding2=[ 138e3 , 0.0, 0.0015 ]  Rm=500  Lm=500  L0=0.5  Saturation=[ 0,0 ; 0.0024,1.2 ; 1.0,1.52 ]  InitialFluxes=[ 0.8 , -0.8 , 0.7 ]  BreakLoop=off  DiscreteSolver=Trapezoidal robust  DataType=off  TransfoNumber=1
      settings: SourceProductName=Simscape Electrical
  T16-18 : powerlib/Elements/Three-Phase Transformer (Two Windings)  Winding1Connection=Delta (D1)  Winding2Connection=Yg  CoreType=Three single-phase transformers  SetSaturation=off  Hysteresis=off  DataFile='hysteresis'  SetInitialFlux=off  Measurements=None  UNITS=pu  NominalPower=[ 10000e6 , 60 ]  Winding1=[ 13.8e3 , 0.0 , 0 ]  Winding2=[ 138e3 , 0.0, 0.003 ]  Rm=500  Lm=500  L0=0.5  Saturation=[ 0,0 ; 0.0024,1.2 ; 1.0,1.52 ]  InitialFluxes=[ 0.8 , -0.8 , 0.7 ]  BreakLoop=off  DiscreteSolver=Trapezoidal robust  DataType=off  TransfoNumber=1
      settings: SourceProductName=Simscape Electrical
  Three-Phase Source : powerlib/Electrical Sources/Three-Phase Source  InternalConnection=Yg  VoltagePhases=off  Voltage=13.8e3  PhaseAngle=0  Voltage_phases=[25e3 25e3 25e3]/sqrt(3)  PhaseAngles_phases=[0 -120 +120]  Frequency=60  NonIdealSource=on  SpecifyImpedance=off  Resistance=0.8929  Inductance=16.58e-3  ShortCircuitLevel=100e6  BaseVoltage=13.8e3  XRratio=7  BusType=PV  Pref=1000e6  Qref=0  Prefabc=[10e3, 10e3, 10e3]  Qrefabc=[0, 0, 0]  Qmin=-inf  Qmax=inf
      settings: SourceProductName=Simscape Electrical
  Three-Phase Source1 : powerlib/Electrical Sources/Three-Phase Source  InternalConnection=Yg  VoltagePhases=off  Voltage=13.8e3  PhaseAngle=0  Voltage_phases=[25e3 25e3 25e3]/sqrt(3)  PhaseAngles_phases=[0 -120 +120]  Frequency=60  NonIdealSource=on  SpecifyImpedance=off  Resistance=0.8929  Inductance=16.58e-3  ShortCircuitLevel=100e6  BaseVoltage=13.8e3  XRratio=7  BusType=swing  Pref=1000e6  Qref=0  Prefabc=[10e3, 10e3, 10e3]  Qrefabc=[0, 0, 0]  Qmin=-inf  Qmax=inf
      settings: SourceProductName=Simscape Electrical
  Three-Phase Source2 : powerlib/Electrical Sources/Three-Phase Source  InternalConnection=Yg  VoltagePhases=off  Voltage=13.8e3  PhaseAngle=0  Voltage_phases=[25e3 25e3 25e3]/sqrt(3)  PhaseAngles_phases=[0 -120 +120]  Frequency=60  NonIdealSource=on  SpecifyImpedance=off  Resistance=0.8929  Inductance=16.58e-3  ShortCircuitLevel=100e6  BaseVoltage=13.8e3  XRratio=7  BusType=PV  Pref=1785e6  Qref=0  Prefabc=[10e3, 10e3, 10e3]  Qrefabc=[0, 0, 0]  Qmin=-inf  Qmax=inf
      settings: SourceProductName=Simscape Electrical
  load18 : powerlib/Elements/Three-Phase Parallel RLC Load  LConnTagsString=A|B|C  Configuration=Y (grounded)  NominalVoltage=138000  Vabc=[1e3 1e3 1e3]  Vabcp=[1e3 1e3 1e3]  NominalFrequency=60  UnbalancedPower=off  ActivePower=2470e6  InductivePower=123e6  CapacitivePower=0  Pabc=[10e3 9e3 11e3]  QLabc=[100 90 110]  QCabc=[100 90 110]  Pabcp=[10e3 9e3 11e3]  QLabcp=[100 90 110]  QCabcp=[100 90 110]  Measurements=None  LoadType=constant PQ
      settings: SourceProductName=Simscape Electrical
  load40 : powerlib/Elements/Three-Phase Parallel RLC Load  LConnTagsString=A|B|C  Configuration=Y (grounded)  NominalVoltage=138000  Vabc=[1e3 1e3 1e3]  Vabcp=[1e3 1e3 1e3]  NominalFrequency=60  UnbalancedPower=off  ActivePower=66e6  InductivePower=24e6  CapacitivePower=0  Pabc=[10e3 9e3 11e3]  QLabc=[100 90 110]  QCabc=[100 90 110]  Pabcp=[10e3 9e3 11e3]  QLabcp=[100 90 110]  QCabcp=[100 90 110]  Measurements=None  LoadType=constant PQ
      settings: SourceProductName=Simscape Electrical
  load41 : powerlib/Elements/Three-Phase Parallel RLC Load  LConnTagsString=A|B|C  Configuration=Y (grounded)  NominalVoltage=138000  Vabc=[1e3 1e3 1e3]  Vabcp=[1e3 1e3 1e3]  NominalFrequency=60  UnbalancedPower=off  ActivePower=1000e6  InductivePower=250e6  CapacitivePower=0  Pabc=[10e3 9e3 11e3]  QLabc=[100 90 110]  QCabc=[100 90 110]  Pabcp=[10e3 9e3 11e3]  QLabcp=[100 90 110]  QCabcp=[100 90 110]  Measurements=None  LoadType=constant PQ
      settings: SourceProductName=Simscape Electrical
  load42 : powerlib/Elements/Three-Phase Parallel RLC Load  LConnTagsString=A|B|C  Configuration=Y (grounded)  NominalVoltage=138000  Vabc=[1e3 1e3 1e3]  Vabcp=[1e3 1e3 1e3]  NominalFrequency=60  UnbalancedPower=off  ActivePower=1150e6  InductivePower=250e6  CapacitivePower=0  Pabc=[10e3 9e3 11e3]  QLabc=[100 90 110]  QCabc=[100 90 110]  Pabcp=[10e3 9e3 11e3]  QLabcp=[100 90 110]  QCabcp=[100 90 110]  Measurements=None  LoadType=constant PQ
      settings: SourceProductName=Simscape Electrical
  load48 : powerlib/Elements/Three-Phase Parallel RLC Load  LConnTagsString=A|B|C  Configuration=Y (grounded)  NominalVoltage=138000  Vabc=[1e3 1e3 1e3]  Vabcp=[1e3 1e3 1e3]  NominalFrequency=60  UnbalancedPower=off  ActivePower=241e6  InductivePower=2e6  CapacitivePower=0  Pabc=[10e3 9e3 11e3]  QLabc=[100 90 110]  QCabc=[100 90 110]  Pabcp=[10e3 9e3 11e3]  QLabcp=[100 90 110]  QCabcp=[100 90 110]  Measurements=None  LoadType=constant PQ
      settings: SourceProductName=Simscape Electrical
  A18 : PMIOPort  Tag=PMCPort  Side=Right
  B18 : PMIOPort  Tag=PMCPort  Port=2  Side=Right
  C18 : PMIOPort  Tag=PMCPort  Port=3  Side=Right
  B48 : PMIOPort  Tag=PMCPort  Port=4  Side=Right
  A48 : PMIOPort  Tag=PMCPort  Port=5  Side=Right
  C48 : PMIOPort  Tag=PMCPort  Port=6  Side=Right
  connections:
  T14-41/LConn3 -- 14/LConn3
  T14-41/LConn2 -- 14/LConn2
  18/LConn1 -- Load Flow Bus5/LConn1 -- load18/LConn1 -- A18/RConn1
  T16-18/LConn2 -- 16/LConn2
  T15-42/LConn3 -- 15/LConn3
  load42/LConn1 -- 19-1/RConn1 -- 42/LConn1 -- Load Flow Bus7/LConn1
  T16-18/LConn3 -- 16/LConn3
  load18/LConn3 -- 18/LConn3 -- C18/RConn1
  48/RConn2 -- 56-1/LConn2
  T14-41/RConn1 -- 41/RConn1
  Three-Phase Source1/RConn3 -- 16/RConn3 -- G16/LConn3
  T15-42/LConn2 -- 15/LConn2
  56-1/RConn3 -- 40/LConn3
  load41/LConn2 -- 55-1/RConn2 -- 41/LConn2 -- 57-1/RConn2
  T14-41/RConn3 -- 41/RConn3
  T14-41/LConn1 -- 14/LConn1
  18/RConn1 -- SSN Interface Block (3ph)/LConn1 -- T16-18/RConn1
  56-1/RConn1 -- 40/LConn1 -- Load Flow Bus3/LConn1
  56-1/RConn2 -- 40/LConn2
  T15-42/LConn1 -- Load Flow Bus1/LConn1 -- 15/LConn1
  Three-Phase Source/RConn1 -- 15/RConn1 -- G15/LConn1
  19-1/RConn2 -- 42/LConn2 -- load42/LConn2
  Three-Phase Source1/RConn1 -- 16/RConn1 -- G16/LConn1
  T16-18/LConn1 -- Load Flow Bus2/LConn1 -- 16/LConn1
  55-1/LConn1 -- load40/LConn1 -- 40/RConn1
  load18/LConn2 -- 18/LConn2 -- B18/RConn1
  18/RConn3 -- SSN group tag1/LConn1 -- SSN Interface Block (3ph)/LConn3 -- T16-18/RConn3
  41/LConn1 -- Load Flow Bus6/LConn1 -- 57-1/RConn1 -- load41/LConn1 -- 55-1/RConn1
  Three-Phase Source2/RConn1 -- Load Flow Bus4/LConn1 -- G14/LConn1 -- 14/RConn1
  Three-Phase Source/RConn3 -- 15/RConn3 -- G15/LConn3
  18/RConn2 -- SSN Interface Block (3ph)/LConn2 -- T16-18/RConn2
  Three-Phase Source2/RConn3 -- 14/RConn3 -- G14/LConn3
  56-1/LConn1 -- 48/RConn1
  Three-Phase Source/RConn2 -- 15/RConn2 -- G15/LConn2
  T15-42/RConn2 -- 42/RConn2 -- 57-1/LConn2
  load41/LConn3 -- 55-1/RConn3 -- 41/LConn3 -- 57-1/RConn3
  48/RConn3 -- 56-1/LConn3
  T15-42/RConn1 -- 42/RConn1 -- 57-1/LConn1
  40/RConn2 -- load40/LConn2 -- 55-1/LConn2
  48/LConn3 -- load48/LConn3 -- C48/RConn1
  Three-Phase Source2/RConn2 -- 14/RConn2 -- G14/LConn2
  T15-42/RConn3 -- 42/RConn3 -- 57-1/LConn3
  19-1/RConn3 -- 42/LConn3 -- load42/LConn3
  Three-Phase Source1/RConn2 -- 16/RConn2 -- G16/LConn2
  40/RConn3 -- load40/LConn3 -- 55-1/LConn3
  A48/RConn1 -- load48/LConn1 -- 48/LConn1 -- Load Flow Bus8/LConn1
  load48/LConn2 -- 48/LConn2 -- B48/RConn1
  T14-41/RConn2 -- 41/RConn2
  SSN Interface Block (3ph)/RConn1 -- 19-1/LConn1
  SSN Interface Block (3ph)/RConn2 -- 19-1/LConn2
  SSN Interface Block (3ph)/RConn3 -- 19-1/LConn3 -- SSN group tag2/LConn1
